simulink model "fxpdemo_filters"  (Simulink 7.6)
settings: Solver=FixedStepDiscrete  SolverMode=SingleTasking  StartTime=0.0  StopTime=1  FixedStep=0.005  RelTol=1e-3  AbsTol=1e-6
InitFcn:
  | ;
StartFcn:
  | ;
StopFcn:
  | ;
undefined symbols (not defined in the file or in its folder): NumBits1, NumBits2, Slope1, Slope2
libraries: fixpt_lib_4 x3, simulink x3
Description:
  | Fixed-Point Filters
  | 
  | Sample bit-true implementations of fixed-point direct type I and II filters with time-varying and
  | time-invariant coefficients are presented.  These filters use the fundamental capabilities in
  | Simulink(R) Fixed Point(TM) and work with the autoscaling tools in Simulink Fixed Point.
  | 
  | Note: the Filter Design Toolbox(TM) and Signal Processing Blockset(TM) leverage this capability and
  | extend it by providing high level design tools and multirate implementations for complex
  | real-time signal processing applications.
PreSaveFcn:
  | ;
CloseFcn:
  | ;
settings Model: MinMaxOverflowLogging=MinMaxAndOverflow  Creator=The MathWorks Inc.  CovMetricSettings=d  ExtModeTrigMode=oneshot  ExtModeArmWhenConnect=off  ExtModeAutoUpdateStatusClock=off
settings DataIOCC: LimitDataPoints=off  SignalLoggingName=sigsOut
settings OptimizationCC: InlineParams=on  InlineInvariantSignals=on  InitFltsAndDblsToZero=on
settings DebuggingCC: SaveWithParameterizedLinksMsg=none  SignalResolutionControl=TryResolveAllWithWarning  SolverPrmCheckMsg=none  MultiTaskDSMMsg=warning  MultiTaskCondExecSysMsg=none  SigSpecEnsureSampleTimeMsg=none  IntegerOverflowMsg=none  ParameterDowncastMsg=warning  ParameterOverflowMsg=warning  ParameterPrecisionLossMsg=none  StrictBusMsg=None
settings HardwareCC: TargetUnknown=on
settings RTWCC: GenerateReport=on  IncludeERTFirstTime=on
settings CodeAppCC: GenerateComments=off  SimulinkBlockComments=off
settings GRTTargetCC: TargetFcnLib=ansi_tfl_tmw.mat

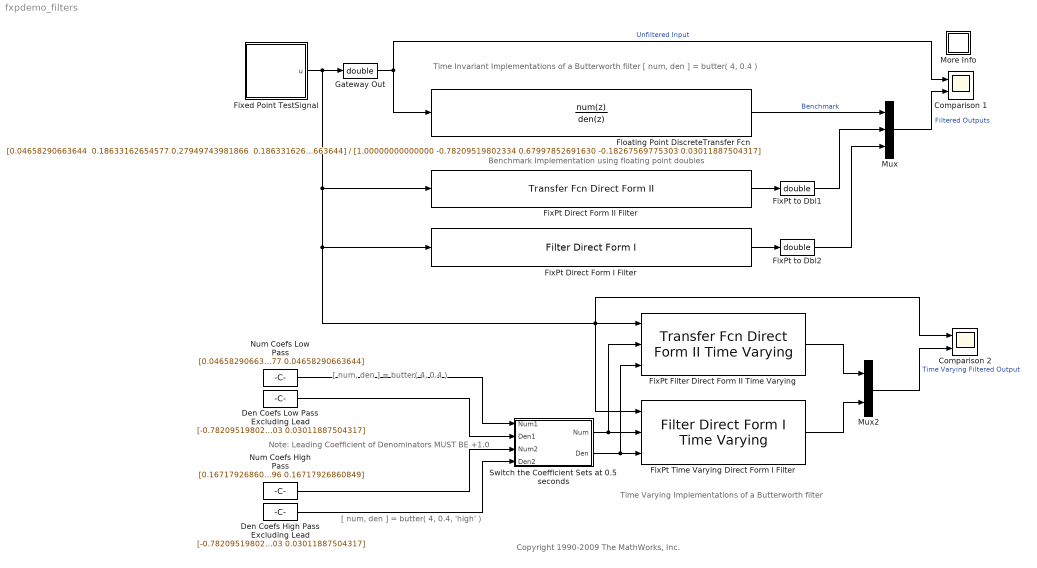
== system fxpdemo_filters ==
  note: Time Invariant
      | Implementations of a Butterworth filter
      | [ num, den ] = butter( 4, 0.4 )
  note: Benchmark Implementation using floating point doubles
  note: Time Varying
      | Implementations of a Butterworth filter
  note: [ num, den ] = butter( 4, 0.4 )
  note: [ num, den ] = butter( 4, 0.4, 'high' )
  note: Note: Leading Coefficient of
      | Denominators MUST BE +1.0
  note: Copyright 1990-2009 The MathWorks, Inc.
  Comparison 1 : Scope  NumInputPorts=2
      settings: TickLabels=on  TimeRange=1  YMin=-1~-0.8  YMax=1~0.6
  Comparison 2 : Scope  NumInputPorts=2
      settings: TickLabels=on  TimeRange=1  YMin=-1~-0.8  YMax=1~0.6  SaveName=ScopeData2
  Den Coefs High Pass Excluding Lead : Constant  Value="[-0.78209519802334   0.67997852691630  -0.18267569775303 0.03011887504317]"  OutDataTypeStr=sfix(16)
  Den Coefs Low Pass Excluding Lead : Constant  Value=[-0.78209519802334 0.67997852691630 -0.18267569775303 0.03011887504317]  OutDataTypeStr=sfix(16)
  FixPt Direct Form I Filter : fixpt_lib_4/Filters/Filter Direct Form I  SystemSampleTime=-1  NumCoefVec="[0.04658290663644  0.18633162654577 0.27949743981866  0.18633162654577 0.04658290663644]"  DenCoefVec=[-0.78209519802334 0.67997852691630 -0.18267569775303 0.03011887504317]  ICPrevOutput=0.0  ICPrevInput=0.0  DoSatur=off
  FixPt Direct Form II Filter : simulink/Additional Math & Discrete/Additional Discrete/Transfer Fcn Direct Form II  SystemSampleTime=-1  NumCoefVec="[0.04658290663644  0.18633162654577 0.27949743981866  0.18633162654577 0.04658290663644]"  DenCoefVec=[-0.78209519802334 0.67997852691630 -0.18267569775303 0.03011887504317]  vinit=0.0  DoSatur=off
  FixPt Filter Direct Form II Time Varying : simulink/Additional Math & Discrete/Additional Discrete/Transfer Fcn Direct Form II Time Varying  SystemSampleTime=-1  vinit=0.0  DoSatur=off
  FixPt Time Varying Direct Form I Filter : fixpt_lib_4/Filters/Filter Direct Form I Time Varying  SystemSampleTime=-1  ICPrevOutput=0.0  ICPrevInput=0.0  DoSatur=off
  FixPt to Dbl1 : DataTypeConversion  OutDataTypeStr=double
  FixPt to Dbl2 : DataTypeConversion  OutDataTypeStr=double
  Fixed Point TestSignal : Subsystem
      mask Display: fprintf('Sine Waves\n0.5 @ 2Hz\nplus\n0.5 @ 80Hz')
  Floating Point DiscreteTransfer Fcn : DiscreteTransferFcn  Numerator="[0.04658290663644  0.18633162654577 0.27949743981866  0.18633162654577 0.04658290663644]"  Denominator=[1.00000000000000 -0.78209519802334 0.67997852691630 -0.18267569775303 0.03011887504317]  SampleTime=-1
  Gateway Out : DataTypeConversion  OutDataTypeStr=double
  More Info : Subsystem
      settings: OpenFcn=showdemo(bdroot(gcs))
      mask Display: disp('?')
  Mux : Mux  Inputs=3
  Mux2 : Mux  Inputs=2
  Num Coefs High Pass : Constant  Value="[0.16717926860849  -0.66871707443396   1.00307561165094  -0.66871707443396 0.16717926860849]"  OutDataTypeStr=sfix(16)
  Num Coefs Low Pass : Constant  Value="[0.04658290663644 0.18633162654577 0.27949743981866  0.18633162654577 0.04658290663644]"  OutDataTypeStr=sfix(16)
  Switch the Coefficient Sets at 0.5 seconds : Subsystem
  wires:
  Fixed Point TestSignal/1(u) -> Gateway Out/1, FixPt Direct Form II Filter/1, Comparison 2/1, FixPt Filter Direct Form II Time Varying/1, FixPt Time Varying Direct Form I Filter/1, FixPt Direct Form I Filter/1
  Floating Point DiscreteTransfer Fcn/1 -> Mux/1  "Benchmark"
  Gateway Out/1 -> Floating Point DiscreteTransfer Fcn/1, Comparison 1/1  "Unfiltered Input"
  Mux2/1 -> Comparison 2/2  "Time Varying Filtered Output"
  FixPt Time Varying Direct Form I Filter/1 -> Mux2/2
  Num Coefs Low Pass/1 -> Switch the Coefficient Sets at 0.5 seconds/1(Num1)
  Den Coefs Low Pass Excluding Lead/1 -> Switch the Coefficient Sets at 0.5 seconds/2(Den1)
  Num Coefs High Pass/1 -> Switch the Coefficient Sets at 0.5 seconds/3(Num2)
  Den Coefs High Pass Excluding Lead/1 -> Switch the Coefficient Sets at 0.5 seconds/4(Den2)
  Switch the Coefficient Sets at 0.5 seconds/1(Num) -> FixPt Filter Direct Form II Time Varying/2, FixPt Time Varying Direct Form I Filter/2
  Switch the Coefficient Sets at 0.5 seconds/2(Den) -> FixPt Filter Direct Form II Time Varying/3, FixPt Time Varying Direct Form I Filter/3
  FixPt Direct Form II Filter/1 -> FixPt to Dbl1/1
  FixPt Direct Form I Filter/1 -> FixPt to Dbl2/1
  FixPt to Dbl1/1 -> Mux/2
  FixPt to Dbl2/1 -> Mux/3
  FixPt Filter Direct Form II Time Varying/1 -> Mux2/1
  Mux/1 -> Comparison 1/2  "Filtered Outputs"

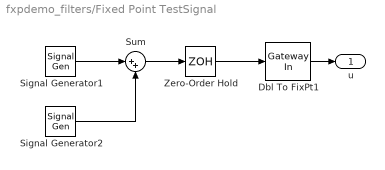
== system fxpdemo_filters/Fixed Point TestSignal ==
  Dbl To FixPt1 : fixpt_lib_4/Data Type/Gateway In  InRealWorld=Real World Value  OutputDataTypeScalingMode=Specify via dialog  OutDataType=sfix(16)  OutScaling=2^(-15)  DoSatur=on
      settings: LockScale=on
  Signal Generator1 : SignalGenerator  Amplitude=0.5  Frequency=2
  Signal Generator2 : SignalGenerator  Amplitude=0.5  Frequency=80
  Sum : Sum  Inputs=|++  SaturateOnIntegerOverflow=on  InputSameDT=on  OutDataTypeStr=Inherit: Same as first input
  Zero-Order Hold : ZeroOrderHold  SampleTime=0.005
  u : Outport
  wires:
  Zero-Order Hold/1 -> Dbl To FixPt1/1
  Sum/1 -> Zero-Order Hold/1
  Signal Generator1/1 -> Sum/1
  Signal Generator2/1 -> Sum/2
  Dbl To FixPt1/1 -> u/1

== system fxpdemo_filters/More Info ==

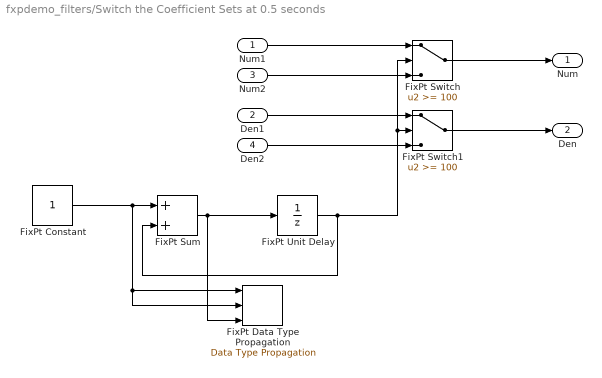
== system fxpdemo_filters/Switch the Coefficient Sets at 0.5 seconds ==
  Num1 : Inport
  Den1 : Inport  Port=2
  Num2 : Inport  Port=3
  Den2 : Inport  Port=4
  FixPt Constant : Constant  OutDataTypeStr=fixdt(0,16,0)
  FixPt Data Type Propagation : simulink/Signal Attributes/Data Type Propagation  PropDataType=sfix(16)  IfRefDouble=double  IfRefSingle=single  IsSigned=IsSigned1 or IsSigned2  NumBitsBase=max([NumBits1 NumBits2])  NumBitsMult=1  NumBitsAdd=0  NumBitsAllowFinal=1:128  PropScaling=2^-10  ValuesUsedBestPrec=[5 -7]  SlopeBase=min([Slope1 Slope2])  SlopeMult=1  SlopeAdd=0  BiasBase=Bias1  BiasMult=1  BiasAdd=0
  FixPt Sum : Sum  OutDataTypeStr=Inherit: Inherit via back propagation
  FixPt Switch : Switch  Threshold=100
  FixPt Switch1 : Switch  Threshold=100
  FixPt Unit Delay : UnitDelay  X0=0.0  SampleTime=-1
  Num : Outport
  Den : Outport  Port=2
  wires:
  FixPt Constant/1 -> FixPt Sum/1, FixPt Data Type Propagation/1, FixPt Data Type Propagation/2
  FixPt Sum/1 -> FixPt Unit Delay/1, FixPt Data Type Propagation/3
  FixPt Unit Delay/1 -> FixPt Sum/2, FixPt Switch/2, FixPt Switch1/2
  Num1/1 -> FixPt Switch/1
  FixPt Switch/1 -> Num/1
  Num2/1 -> FixPt Switch/3
  Den1/1 -> FixPt Switch1/1
  FixPt Switch1/1 -> Den/1
  Den2/1 -> FixPt Switch1/3
